simulink model "punto2"  (R2017b)
settings: Solver=VariableStepAuto  StartTime=0.0  StopTime=.3  RelTol=1e-3
values from neighbouring files (symbols this model uses):
  f = 1.86*10^-3    (= 0.00186)    [Practica5.m]    (also in punto1.m)
  Kem = 0.67    [Practica5.m]    (also in punto1.m)
  p1 = nd(2)*q0    [Practica5.m]    (also in punto1.m)
  p2 = nd(3)*q0    [Practica5.m]    (also in punto1.m)
  q0 = 1/sum(nd)    [Practica5.m]    (also in punto1.m)
  q1 = dd(2)*q0    [Practica5.m]    (also in punto1.m)
  q2 = dd(3)*q0    [Practica5.m]    (also in punto1.m)
  R = 8    [Practica5.m]    (also in punto1.m)
  T0 = .5    (= 0.5)    [Practica5.m]    (also in punto1.m = 0.02)
  Tcarga = 0.1    [Practica5.m]    (also in punto1.m)
  Te = L/R    (= 0.01)    [Practica5.m]    (also in punto1.m)
  Tm = J/f    (= 1.1935483871)    [Practica5.m]    (also in punto1.m)
settings Model: Creator=Agustin  LastModifiedBy=Agustin

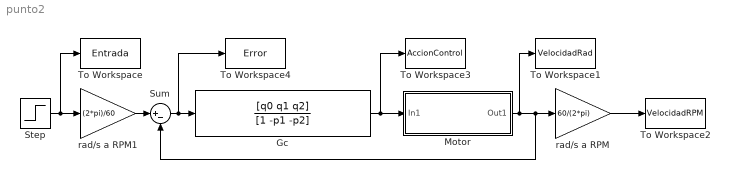
== system punto2 ==
  Gc : DiscreteTransferFcn  Numerator=[q0 q1 q2]  Denominator=[1 -p1 -p2]  SampleTime=T0
  Motor : Subsystem
  Step : Step  Time=0  After=1000  SampleTime=0
  Sum : Sum  Inputs=|+-
  To Workspace : ToWorkspace  VariableName=Entrada  SaveFormat=Timeseries  SampleTime=-1
  To Workspace1 : ToWorkspace  VariableName=VelocidadRad  SaveFormat=Timeseries  SampleTime=-1
  To Workspace2 : ToWorkspace  VariableName=VelocidadRPM  SaveFormat=Timeseries  SampleTime=-1
  To Workspace3 : ToWorkspace  VariableName=AccionControl  SaveFormat=Timeseries  SampleTime=-1
  To Workspace4 : ToWorkspace  VariableName=Error  SaveFormat=Timeseries  SampleTime=-1
  rad/s a RPM : Gain  Gain=60/(2*pi)
  rad/s a RPM1 : Gain  Gain=(2*pi)/60
  wires:
  Motor/1(Out1) -> To Workspace1/1, Sum/2, rad/s a RPM/1
  rad/s a RPM/1 -> To Workspace2/1
  Step/1 -> To Workspace/1, rad/s a RPM1/1
  Gc/1 -> To Workspace3/1, Motor/1(In1)
  Sum/1 -> To Workspace4/1, Gc/1
  rad/s a RPM1/1 -> Sum/1

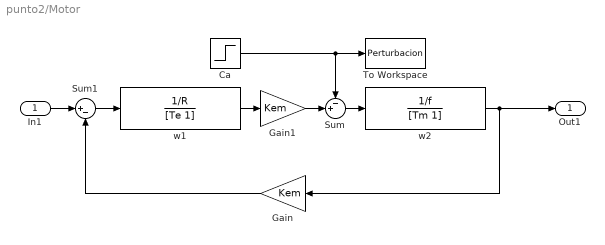
== system punto2/Motor ==
  In1 : Inport
  Ca : Step  Time=Tcarga  After=2  SampleTime=0
  Gain : Gain  Gain=Kem
  Gain1 : Gain  Gain=Kem
  Sum : Sum  Inputs=-+|
  Sum1 : Sum  Inputs=|+-
  To Workspace : ToWorkspace  VariableName=Perturbacion  SaveFormat=Timeseries  SampleTime=-1
  w1 : TransferFcn  Numerator=1/R  Denominator=[Te 1]
  w2 : TransferFcn  Numerator=1/f  Denominator=[Tm 1]
  Out1 : Outport
  wires:
  w2/1 -> Out1/1, Gain/1
  Sum/1 -> w2/1
  Ca/1 -> To Workspace/1, Sum/1
  Gain1/1 -> Sum/2
  w1/1 -> Gain1/1
  Gain/1 -> Sum1/2
  In1/1 -> Sum1/1
  Sum1/1 -> w1/1
